simulink model "aerotesthigh"  (Simulink 5.0)
settings: Solver=ode1  SolverMode=SingleTasking  StartTime=0.0  StopTime=150  FixedStep=1  RelTol=1e-3  AbsTol=1e-6
libraries: simulink x1
settings Model: Creator=hkg  LastModifiedBy=hkg  ModifiedComment=nnt -- Mon Jun 05 13:08:11 2000 -- Version 3.42  ExtModeTrigMode=oneshot  ExtModeArmWhenConnect=off  SaveState=on  LimitDataPoints=off  ConsistencyChecking=warning  BooleanDataType=off  RTWTemplateMakefile=grt_adm5p3.tmf  RTWOptions="-aLogVarNameModifier=\"rt_\" -aExtMode=0 -aRollThreshold=5 -aShowEliminatedStatements=1 -aRTWVerbose=1 -aInlineInvariantSignals=1 -aLocalBlockOutputs=1 -aInlineParameters=0"
settings Model: ModifiedHistory=|
  | nnt -- Mon Jun 05 13:08:11 2000 -- Version 3.42
  | 
  | 
  | nnt -- Mon Jun 05 11:01:33 2000 -- Version 3.41
  | 
  | 
  | nnt -- Mon Jun 05 10:57:40 2000 -- Version 3.40
  | 
  | 
  | nnt -- Mon Jun 05 10:56:46 2000 -- Version 3.39
  | 
  | 
  | hkg -- Thu Apr 13 16:38:30 2000 -- Version 3.38
  | Bug fix: all rate limiters were set with the canard parameters, now they get individual settings..
  | 
  | hkg -- Thu Apr 13 10:24:31 2000 -- Version 3.37
  | Inserted 3.0 version number in Level 1, changed month to April.
  | 
  | hkg -- Tue Apr 11 10:36:55 2000 -- Version 3.36
  | dtz re-connected
  | 
  | hkg -- Tue Apr 11 10:28:52 2000 -- Version 3.35
  | Changed the roll force saturation to +-80 N
  | 
  | hkg -- Tue Apr 11 09:23:02 2000 -- Version 3.34
  | All signal generators on Level 1 are now set to sine wave
  | 
  | hkg -- Mon Apr 10 15:03:16 2000 -- Version 3.33
  | New names for the RL_choice blocks
  | 
  | fosimadmin -- Mon Apr 10 13:44:14 2000 -- Version 3.32
  | Hkg actually. Nothing special
  | 
  | hkg -- Fri Apr 07 14:32:16 2000 -- Version 3.31
  | A few corrections to the names
  | 
  | hkg -- Fri Apr 07 14:16:55 2000 -- Version 3.30
  | Added unique names inside Saab and DASA rate limiters for left elevons, rudder and
  | leading-edge flaps.
  | hkg -- Fri Apr 07 14:04:35 2000 -- Version 3.29
  | Added unique names inside SAAB and DASA rate limiters for canard and right outer and
  | inner elevons.
  | hkg -- Thu Apr 06 17:23:24 2000 -- Version 3.28
  | Inserted unique names for rate limiters and multiport switches in the rate limiter selection blocks.
  | hkg -- Thu Apr 06 16:09:22 2000 -- Version 3.27
  | Disconnected dtz again. Chosen grt_adm5p3.tmf as template makefile. Code generation seems to work.
  | hyd -- Tue Mar 28 15:20:39 2000 -- Version 3.26
  | hyd -- Tue Mar 28 14:28:32 2000 -- Version 3.25
  | hyd -- Tue Mar 28 11:30:24 2000 -- Version 3.24
  | hyd -- Mon Mar 27 15:22:27 2000 -- Version 3.23
  | hyd -- Mon Mar 27 13:42:12 2000 -- Version 3.22
  | hyd -- Mon Mar 27 10:51:54 2000 -- Version 3.21
  | hyd -- Fri Mar 24 13:18:05 2000 -- Version 3.20
  | hyd -- Fri Mar 24 12:50:02 2000 -- Version 3.19
  | hyd -- Fri Mar 24 11:54:23 2000 -- Version 3.18
  | hyd -- Thu Mar 23 15:20:42 2000 -- Version 3.17
  | hyd -- Thu Mar 23 15:17:54 2000 -- Version 3.16
  | hyd -- Wed Mar 22 09:38:49 2000 -- Version 3.15
  | hyd -- Tue Mar 21 14:06:08 2000 -- Version 3.14
  | hyd -- Mon Mar 20 14:42:54 2000 -- Version 3.13
  | hyd -- Wed Mar 15 13:37:48 2000 -- Version 3.12
  | hyd -- Wed Mar 15 12:35:54 2000 -- Version 3.11
  | jnr -- Tue Mar 14 16:36:26 2000 -- Version 3.10
  | jnr -- Tue Mar 14 14:13:39 2000 -- Version 3.9
  | jnr -- Tue Mar 14 14:13:23 2000 -- Version 3.8
  | jnr -- Tue Mar 14 10:09:15 2000 -- Version 3.7
  | jnr -- Tue Mar 14 09:37:34 2000 -- Version 3.6
  | jnr -- Tue Mar 14 09:30:20 2000 -- Version 3.5
  | Add:
  | *proper stick gradients.
  | *correct gains for nz-control according to Åke Hydén.
  | *what transition region between q-control and nz-control is proper??
  | fll -- Fri Mar 03 09:53:48 2000 -- Version 3.4
  | changed name of "dtx" to "dty" (horizontal nozzle deflection)
  | fll -- Thu Mar 02 12:51:23 2000 -- Version 3.3
  | Reducesed the number of integrators to one in the longitudinal controller.
  | fll -- Thu Mar 02 12:30:52 2000 -- Version 3.2
  | Moved the blending function in the Nz and q controller.
  | fll -- Thu Mar 02 10:50:25 2000 -- Version 3.1
  | Changed input blocks to "Signal generator"
  | fll -- Thu Mar 02 10:50:25 2000 -- Version 3.0
  | Version 3.0 is modified according to comments from users

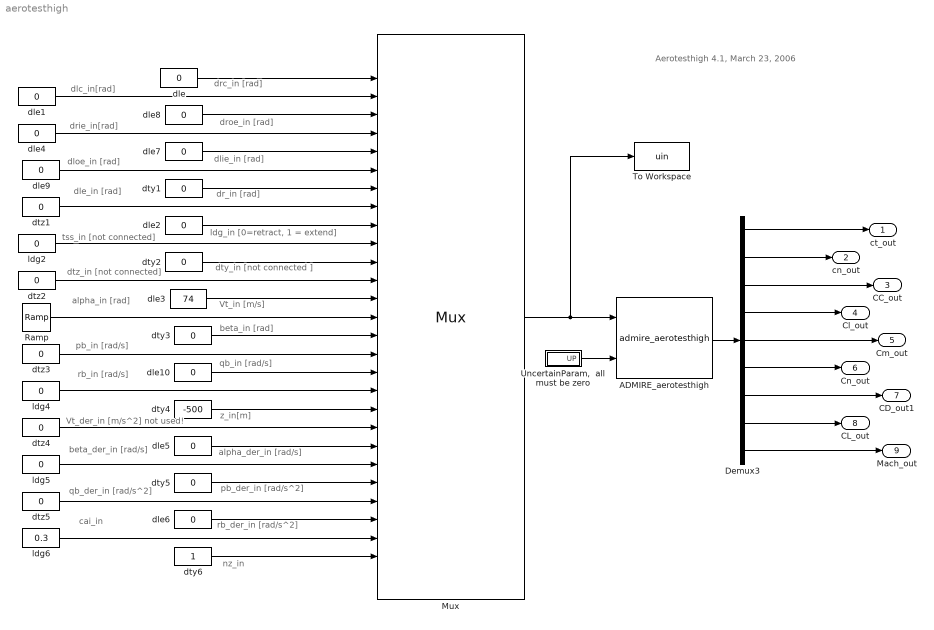
== system aerotesthigh ==
  note: drc_in [rad]
  note: dlc_in[rad]
  note: droe_in [rad]
  note: drie_in[rad]
  note: dlie_in [rad]
  note: dloe_in [rad]
  note: dr_in [rad]
  note: dle_in [rad]
  note: ldg_in [0=retract, 1 = extend]
  note: tss_in [not connected]
  note: dty_in [not connected ]
  note: Vt_in [m/s]
  note: alpha_in [rad]
  note: pb_in [rad/s]
  note: rb_in [rad/s]
  note: z_in[m]
  note: Vt_der_in [m/s^2] not used!
  note: alpha_der_in [rad/s]
  note: beta_der_in [rad/s]
  note: pb_der_in [rad/s^2]
  note: qb_der_in [rad/s^2]
  note: rb_der_in [rad/s^2]
  note: cai_in
  note: nz_in
  note: dtz_in [not connected]
  note: qb_in [rad/s]
  note: beta_in [rad]
  note: Aerotesthigh 4.1, March 23, 2006
  ADMIRE_aerotesthigh : S-Function  FunctionName=admire_aerotesthigh
      mask Type: ADMIRE C-code block
      mask Description:
      | Main block describing the ADMIRE.
      | To use HELP, start any Internet browser.
      mask Help:
      | The aircraft it self is a C-code file that calculates the dynamics of the structure and the air surrounding it.<br>
      | The simulation requires an initial vector of values called x0 containing the following variables.<br><br>
      | 
      | Vt_init     --     initial airspeed.                        [m/s]<br>
      | alpha_init --    initial angle of attack.             [rad]<br>
      | beta_init    --   initial angle of sideslip.            [rad]<br>
      | pb_init     --     initial roll angular rate.             [rad/s]<br>
      | qb_init     --     initial pitch angular rate.          [rad/s]<br>
      | rb_init       --    initial yaw angular rate.           [rad/s]<br>
      | psi_init      --    initial euler angles (azimuth)    [rad]<br>
      | theta_init   --   initial (elevation)                      [rad]<br>
      | phi_init      --   initial (bank)                             [rad]<br>
      | xv_init      --    initial x position in Fv                [m]<br>
      | yv_init        --  initial y                                     [m]<br>
      | zv_init       --   initial z                                     [m]<br>
      mask Display:
      | plot([18 12 3 2 2 8 11],[7 4 1 1 2 8 11])
      | plot([13 11 13 15 15 13],[12 11 16 17 13 12])
      | plot([15 17 20 23 30 17],[13 14 24 25 20 14])
      | plot([30 38 40 38 30],[19 31 32 22 19])
      | plot([38.5 41 36 22 41 43 36],[23 21 16 10 8 10 16])
      | plot([15 19 25 24 15],[7 9 9 8 7])
      | plot([8 11 13 14 9 8],[8 11 12 10 7 8])
      | plot([21 23],[9 10])
      | plot([30 31],[20 20.5])
  Demux3 : Demux  Outputs=9
  Mux : Mux  Inputs=27
      settings: DisplayOption=signals
  Ramp : simulink/Sources/Ramp  slope=125*pi/180/100  start=0  X0=-35*pi/180
  To Workspace : ToWorkspace  VariableName=uin  SampleTime=-1  SaveFormat=Array
  "UncertainParam,  all must be zero" : Subsystem
      mask Display: plot([0 10 5 0],[0 0 8.6603 0])
  dle{,1..2,4..10} (10 alike) : Constant  Value=0
  dle3 : Constant  Value=74
  dty{1..3,5} (4 alike) : Constant  Value=0
  dty4 : Constant  Value=-500
  dty6 : Constant
  dtz{1..5} (5 alike) : Constant  Value=0
  ldg2 : Constant  Value=0
  ldg4 : Constant  Value=0
  ldg5 : Constant  Value=0
  ldg6 : Constant  Value=0.3
  ct_out : Outport
  cn_out : Outport  Port=2
  CC_out : Outport  Port=3
  Cl_out : Outport  Port=4
  Cm_out : Outport  Port=5
  Cn_out : Outport  Port=6
  CD_out1 : Outport  Port=7
  CL_out : Outport  Port=8
  Mach_out : Outport  Port=9
  wires:
  dle2/1 -> Mux/9
  dty2/1 -> Mux/11
  dle1/1 -> Mux/2
  dle4/1 -> Mux/4
  dle9/1 -> Mux/6
  dtz1/1 -> Mux/8
  ldg2/1 -> Mux/10
  ldg4/1 -> Mux/18
  dtz4/1 -> Mux/20
  ldg5/1 -> Mux/22
  dtz5/1 -> Mux/24
  ldg6/1 -> Mux/26
  dle/1 -> Mux/1
  dle7/1 -> Mux/5
  dty1/1 -> Mux/7
  dle3/1 -> Mux/13
  dle10/1 -> Mux/17
  dty4/1 -> Mux/19
  dle5/1 -> Mux/21
  dty5/1 -> Mux/23
  dle6/1 -> Mux/25
  dty6/1 -> Mux/27
  "UncertainParam,  all must be zero"/1(UP) -> ADMIRE_aerotesthigh/2
  Mux/1 -> ADMIRE_aerotesthigh/1, To Workspace/1
  dtz3/1 -> Mux/16
  dty3/1 -> Mux/15
  dle8/1 -> Mux/3
  Ramp/1 -> Mux/14
  ADMIRE_aerotesthigh/1 -> Demux3/1
  Demux3/2 -> cn_out/1
  Demux3/4 -> Cl_out/1
  Demux3/6 -> Cn_out/1
  Demux3/5 -> Cm_out/1
  Demux3/1 -> ct_out/1
  Demux3/3 -> CC_out/1
  Demux3/7 -> CD_out1/1
  Demux3/8 -> CL_out/1
  Demux3/9 -> Mach_out/1
  dtz2/1 -> Mux/12

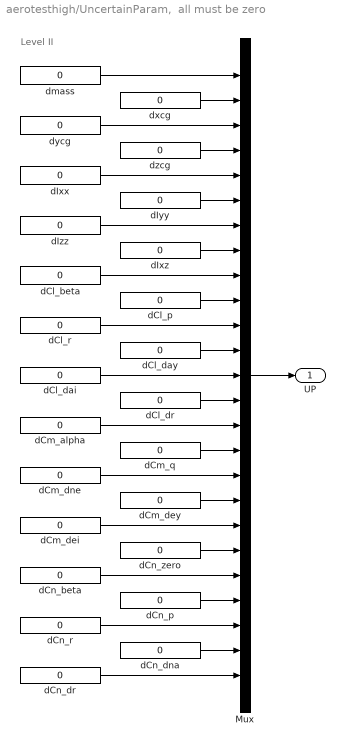
== system aerotesthigh/UncertainParam,  all must be zero ==
  note: Level II
  Mux : Mux  Inputs=25
  "dCl_beta " : Constant  Value=0
  "dCl_dai " : Constant  Value=0
  dCl_day : Constant  Value=0
  "dCl_dr " : Constant  Value=0
  "dCl_p " : Constant  Value=0
  "dCl_r " : Constant  Value=0
  "dCm_alpha " : Constant  Value=0
  "dCm_dei " : Constant  Value=0
  "dCm_dey " : Constant  Value=0
  "dCm_dne " : Constant  Value=0
  "dCm_q " : Constant  Value=0
  "dCn_beta " : Constant  Value=0
  dCn_dna : Constant  Value=0
  "dCn_dr " : Constant  Value=0
  "dCn_p " : Constant  Value=0
  "dCn_r " : Constant  Value=0
  dCn_zero : Constant  Value=0
  dIxx : Constant  Value=0
  dIxz : Constant  Value=0
  "dIyy " : Constant  Value=0
  "dIzz " : Constant  Value=0
  "dmass " : Constant  Value=0
  dxcg : Constant  Value=0
  "dycg " : Constant  Value=0
  "dzcg " : Constant  Value=0
  UP : Outport  InitialOutput=0
  wires:
  dCn_dna/1 -> Mux/24
  "dmass "/1 -> Mux/1
  "dycg "/1 -> Mux/3
  dxcg/1 -> Mux/2
  "dzcg "/1 -> Mux/4
  dIxx/1 -> Mux/5
  "dIyy "/1 -> Mux/6
  "dIzz "/1 -> Mux/7
  dIxz/1 -> Mux/8
  "dCl_beta "/1 -> Mux/9
  "dCl_p "/1 -> Mux/10
  "dCl_r "/1 -> Mux/11
  dCl_day/1 -> Mux/12
  "dCl_dai "/1 -> Mux/13
  "dCl_dr "/1 -> Mux/14
  "dCm_alpha "/1 -> Mux/15
  "dCm_q "/1 -> Mux/16
  "dCm_dey "/1 -> Mux/18
  dCn_zero/1 -> Mux/20
  "dCn_p "/1 -> Mux/22
  Mux/1 -> UP/1
  "dCm_dne "/1 -> Mux/17
  "dCm_dei "/1 -> Mux/19
  "dCn_beta "/1 -> Mux/21
  "dCn_dr "/1 -> Mux/25
  "dCn_r "/1 -> Mux/23
